simulink model "MBD_FOC_HOST"  (R2022b)
settings: Solver=FixedStepDiscrete  StartTime=0.0  StopTime=Inf  RelTol=1e-3
libraries: instrumentseriallib x3
settings Model: Creator=The MathWorks, Inc.  LastModifiedBy=Administrator
settings SolverCC: AlgebraicLoopSolver=TrustRegion  MaxZcPerStep=1
settings DebuggingCC: ParameterPrecisionLossMsg=none  UnconnectedInputMsg=warning  UnconnectedOutputMsg=warning  UnconnectedLineMsg=warning  SFMachineParentedDataDiag=warning
settings ModelReferenceCC: EnableRefExpFcnMdlSchedulingChecks=on
settings RTWCC: DLArmComputeVersion=19.05

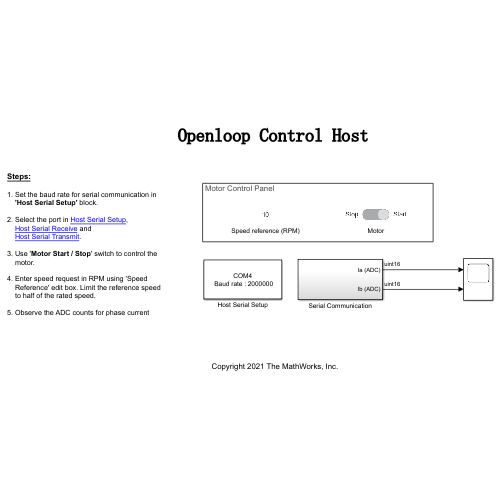
[thumbnail: Simulink's stored preview of the top-level diagram]
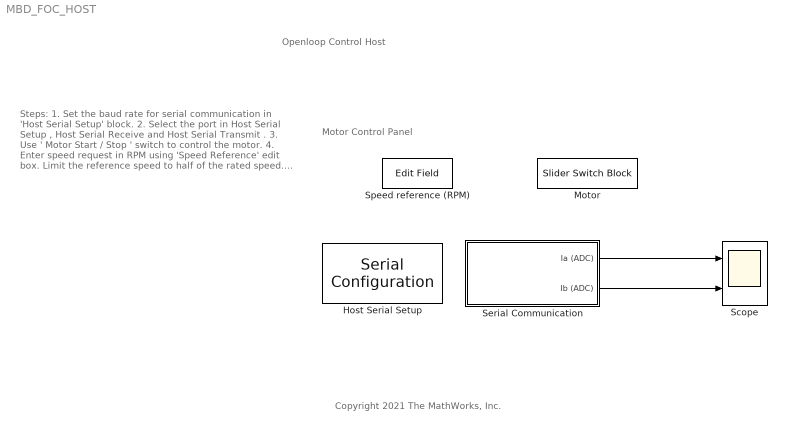
== system MBD_FOC_HOST ==
  note: Openloop Control Host
  note: Copyright 2021 The MathWorks, Inc.
  note: Steps:
      |
      | 1. Set the baud rate for serial communication in
      | 'Host Serial Setup' block.
      |
      | 2. Select the port in Host Serial Setup ,
      | Host Serial Receive and
      | Host Serial Transmit .
      |
      | 3. Use ' Motor Start / Stop ' switch to control the
      | motor.
      |
      | 4. Enter speed request in RPM using 'Speed
      | Reference' edit box. Limit the reference speed
      | to half of the rated speed.
      |
      | 5. Observe the ADC counts for phase current measurent in Scope.
  note: Motor Control Panel
  Host Serial Setup : instrumentseriallib/Serial Configuration  Priority=-99  PortSel=COM4  Port=COM4  ComPort=COM4  BaudRate=2000000  DataBits=8  Parity=none  StopBits=1  ByteOrder=little-endian  FlowControl=none  Timeout=2.0  SimulateUsing=Interpreted execution  BlockInModel=on  aMode=5
  Motor : SliderSwitchBlock  LabelPosition=Hide
      settings: Values={{'Stop', 'Start'}, [0 1]}
  Scope : Scope  NumInputPorts=2
  Serial Communication : Subsystem
  Speed reference (RPM) : EditField  LabelPosition=Hide  ShowInitialText=on  Alignment=Center
  wires:
  Serial Communication/1(Ia (ADC)) -> Scope/1
  Serial Communication/2(Ib (ADC)) -> Scope/2

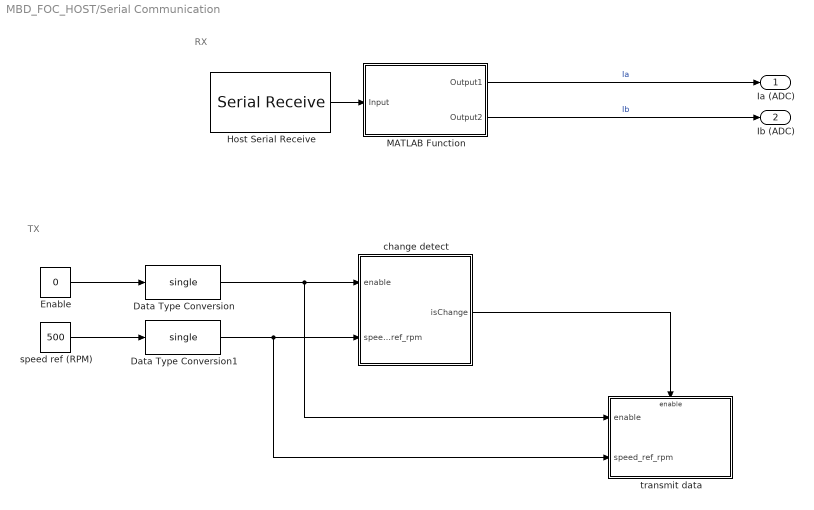
== system MBD_FOC_HOST/Serial Communication ==
  note: TX
  note: RX
  Data Type Conversion : DataTypeConversion  OutDataTypeStr=single  SaturateOnIntegerOverflow=off  RndMeth=Floor
  Data Type Conversion1 : DataTypeConversion  OutDataTypeStr=single  SaturateOnIntegerOverflow=off  RndMeth=Floor  LockScale=on
  Enable : Constant  Value=0  OutDataTypeStr=boolean  SampleTime=-1
  Host Serial Receive : instrumentseriallib/Serial Receive  PortSel=COM4  Port=COM4  ComPort=COM4  DataType=uint16  SaveDataType=uint8  ToggleHeader=on  Header='ss'  ToggleTerminator=on  Terminator=Custom terminator  CustomTerminator='ee'  InputFormat=Row major  ToggleDataSize=on  DataSize=[200 2]  EnableBlockingMode=on  ActionDataUnavailable=Output custom value  ActionWhenDataUnavailable=Output custom value  CustomValue=4000  SampleTime=200 * 50e-6  SimulateUsing=Interpreted execution  BlockInModel=on  aMode=5
  MATLAB Function : MATLAB Function  TreatAsAtomicUnit=on
  change detect : Subsystem
  speed ref (RPM) : Constant  Value=500  OutDataTypeStr=single  SampleTime=-1
  transmit data : Subsystem  TreatAsAtomicUnit=on
  Ia (ADC) : Outport
  Ib (ADC) : Outport  Port=2
  wires:
  Host Serial Receive/1 -> MATLAB Function/1(Input)
  MATLAB Function/1(Output1) -> Ia (ADC)/1  "Ia"
  MATLAB Function/2(Output2) -> Ib (ADC)/1  "Ib"
  Data Type Conversion1/1 -> transmit data/2(speed_ref_rpm), change detect/2(speed_ref_rpm)
  Data Type Conversion/1 -> transmit data/1(enable), change detect/1(enable)
  change detect/1(isChange) -> transmit data/Enable
  speed ref (RPM)/1 -> Data Type Conversion1/1
  Enable/1 -> Data Type Conversion/1

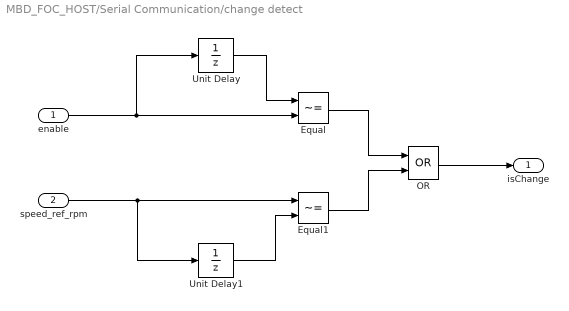
== system MBD_FOC_HOST/Serial Communication/change detect ==
  enable : Inport
  speed_ref_rpm : Inport  Port=2
  Equal : RelationalOperator  Operator=~=  OutDataTypeStr=boolean  RndMeth=Simplest  InputSameDT=off
  Equal1 : RelationalOperator  Operator=~=  OutDataTypeStr=boolean  RndMeth=Simplest  InputSameDT=off
  OR : Logic  Operator=OR  AllPortsSameDT=off  OutDataTypeStr=boolean
  Unit Delay : UnitDelay  SampleTime=-1  HasFrameUpgradeWarning=on
  Unit Delay1 : UnitDelay  SampleTime=-1  HasFrameUpgradeWarning=on
  isChange : Outport
  wires:
  Unit Delay/1 -> Equal/1
  enable/1 -> Equal/2, Unit Delay/1
  speed_ref_rpm/1 -> Unit Delay1/1, Equal1/1
  Unit Delay1/1 -> Equal1/2
  OR/1 -> isChange/1
  Equal/1 -> OR/1
  Equal1/1 -> OR/2

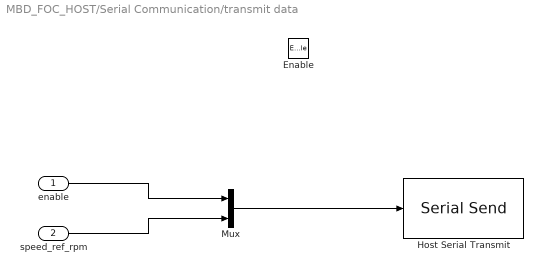
== system MBD_FOC_HOST/Serial Communication/transmit data ==
  enable : Inport
  speed_ref_rpm : Inport  Port=2
  Enable : EnablePort
  Host Serial Transmit : instrumentseriallib/Serial Send  PortSel=COM4  Port=COM4  ComPort=COM4  Header=[]  Terminator=<none>  CustomTerminator=[]  EnableBlockingMode=off  SimulateUsing=Interpreted execution  BlockInModel=on  aMode=5
  Mux : Mux  Inputs=2
  wires:
  enable/1 -> Mux/1
  speed_ref_rpm/1 -> Mux/2
  Mux/1 -> Host Serial Transmit/1

== matlab function MBD_FOC_HOST/Serial Communication/MATLAB Function ==
  data: Output1 output; Output2 output; Input input
function [ Output1, Output2] = unBuf(Input)

Output1 = Input(:, 1);
Output2 = Input(:, 2);
end
